simulink model "dynsim_edo"  (R2020a)
settings: Solver=ode3  StartTime=0.0  StopTime=10.0  FixedStep=0.001  RelTol=1e-3
model workspace (MAT data in the model file):
  SL_ROS_VariableLengthArrays_MaxSizes.CommonInfo.ArrayTruncateAction = 'EmitWarning'
  SL_ROS_VariableLengthArrays_MaxSizes.MsgTypeMap = containers.Map
  SL_ROS_VariableLengthArrays_MaxSizes.MsgTypeMap.serialization.keys = {}
  SL_ROS_VariableLengthArrays_MaxSizes.MsgTypeMap.serialization.values = {}
  SL_ROS_VariableLengthArrays_MaxSizes.MsgTypeMap.serialization.uniformity = 0
  SL_ROS_VariableLengthArrays_MaxSizes.MsgTypeMap.serialization.keyType = 'char'
  SL_ROS_VariableLengthArrays_MaxSizes.MsgTypeMap.serialization.valueType = 'any'
values from neighbouring files (symbols this model uses):
  L1 = 1    [init_edo.m]
  L2 = 1    [init_edo.m]
  L3 = 1    [init_edo.m]
  L4 = 1    [init_edo.m]
  L5 = 1    [init_edo.m]
  L6 = 1    [init_edo.m]
libraries: robotlib x18, robotmaniplib x1
settings Model: Creator=bascetta  LastModifiedBy=davide
settings OptimizationCC: EnhancedBackFolding=on  PassReuseOutputArgsAs=Individual arguments  ZeroExternalMemoryAtStartup=off  ZeroInternalMemoryAtStartup=off  MaxStackSize=64  OptimizeBlockOrder=speed  DifferentSizesBufferReuse=on  OptimizationCustomize=off  EfficientTunableParamExpr=on
settings DebuggingCC: ParameterTunabilityLossMsg=error
settings HardwareCC: ProdBitPerPointer=32  ProdBitPerSizeT=32  ProdBitPerPtrDiffT=32  ProdLargestAtomicFloat=None  ProdIntDivRoundTo=Undefined  ProdEndianess=Unspecified  ProdWordSize=32  ProdHWDeviceType=Generic->Unspecified (assume 32-bit Generic)
settings RTWCC: SystemTargetFile=ert.tlc  HardwareBoard=Robot Operating System (ROS)  TemplateMakefile=ert_default_tmf  GenerateReport=on  Toolchain=Catkin  IncludeHyperlinkInReport=on  LaunchReport=on  TargetLang=C++  GenerateTraceInfo=on  GenerateTraceReport=on  GenerateTraceReportSl=on  GenerateTraceReportSf=on  GenerateTraceReportEml=on
settings CodeAppCC: ForceParamTrailComments=on  IgnoreCustomStorageClasses=off  OperatorAnnotations=on  SimulinkDataObjDesc=on  SFDataObjDesc=on  InsertBlockDesc=on
settings ERTTargetCC: SupportContinuousTime=on  SupportVariableSizeSignals=on

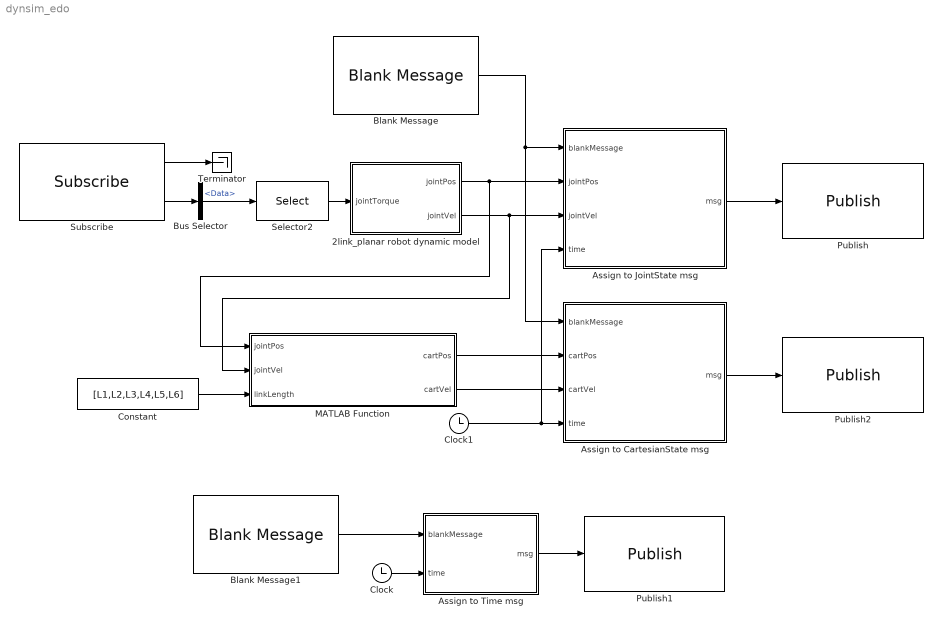
== system dynsim_edo ==
  2link_planar robot dynamic model : Subsystem
  Assign to CartesianState msg : MATLAB Function  TreatAsAtomicUnit=on
  Assign to JointState msg : MATLAB Function  TreatAsAtomicUnit=on
  Assign to Time msg : MATLAB Function  TreatAsAtomicUnit=on
  Blank Message : robotlib/Blank Message  messageClass=Message  entityType=sensor_msgs/JointState  messageType=sensor_msgs/JointState  SampleTime=inf
  Blank Message1 : robotlib/Blank Message  messageClass=Message  entityType=rosgraph_msgs/Clock  messageType=rosgraph_msgs/Clock  SampleTime=inf
  Bus Selector : BusSelector  OutputSignals=Data
  Clock : Clock
  Clock1 : Clock
  Constant : Constant  Value=[L1,L2,L3,L4,L5,L6]
  MATLAB Function : MATLAB Function  TreatAsAtomicUnit=on
  Publish : robotlib/Publish  topicSource=Specify your own  topic=/joint_states  messageType=sensor_msgs/JointState  messageQueueLength=1
  Publish1 : robotlib/Publish  topicSource=Specify your own  topic=/clock  messageType=rosgraph_msgs/Clock  messageQueueLength=1
  Publish2 : robotlib/Publish  topicSource=Specify your own  topic=/cartesian_states  messageType=sensor_msgs/JointState  messageQueueLength=1
  Selector2 : Selector  IndexOptions=Starting index (dialog)  Indices=[2]  OutputSizes=6
  Subscribe : robotlib/Subscribe  topicSource=Specify your own  topic=/joint_torque  messageType=std_msgs/Float64MultiArray  sampleTime=-1  messageQueueLength=1
  Terminator : Terminator
  wires:
  Blank Message1/1 -> Assign to Time msg/1(blankMessage)
  Assign to Time msg/1(msg) -> Publish1/1
  Subscribe/2 -> Bus Selector/1
  Subscribe/1 -> Terminator/1
  Selector2/1 -> 2link_planar robot dynamic model/1(jointTorque)
  Assign to JointState msg/1(msg) -> Publish/1
  2link_planar robot dynamic model/2(jointVel) -> MATLAB Function/2(jointVel), Assign to JointState msg/3(jointVel)
  Bus Selector/1 -> Selector2/1  "<Data>"
  2link_planar robot dynamic model/1(jointPos) -> MATLAB Function/1(jointPos), Assign to JointState msg/2(jointPos)
  Clock/1 -> Assign to Time msg/2(time)
  Clock1/1 -> Assign to CartesianState msg/4(time), Assign to JointState msg/4(time)
  MATLAB Function/2(cartVel) -> Assign to CartesianState msg/3(cartVel)
  Assign to CartesianState msg/1(msg) -> Publish2/1
  Constant/1 -> MATLAB Function/3(linkLength)
  MATLAB Function/1(cartPos) -> Assign to CartesianState msg/2(cartPos)
  Blank Message/1 -> Assign to CartesianState msg/1(blankMessage), Assign to JointState msg/1(blankMessage)

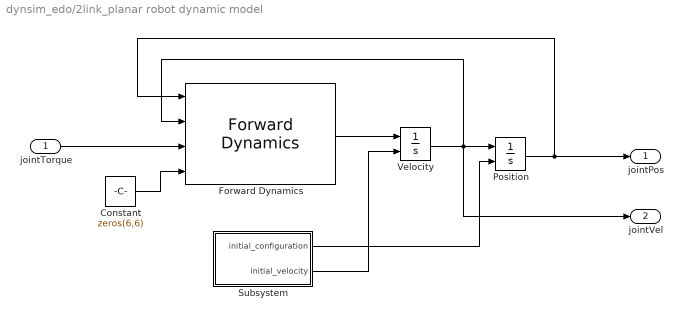
== system dynsim_edo/2link_planar robot dynamic model ==
  jointTorque : Inport
  Constant : Constant  Value=zeros(6,6)
  Forward Dynamics : robotmaniplib/Forward Dynamics  RigidBodyTree=robot_edo  SimulateUsing=Interpreted execution
  Position : Integrator  InitialConditionSource=external
  Subsystem : Subsystem
  Velocity : Integrator  InitialConditionSource=external
  jointPos : Outport
  jointVel : Outport  Port=2
  wires:
  Forward Dynamics/1 -> Velocity/1
  Position/1 -> Forward Dynamics/1, jointPos/1
  jointTorque/1 -> Forward Dynamics/3
  Constant/1 -> Forward Dynamics/4
  Velocity/1 -> Forward Dynamics/2, Position/1, jointVel/1
  Subsystem/2(initial_velocity) -> Velocity/2
  Subsystem/1(initial_configuration) -> Position/2

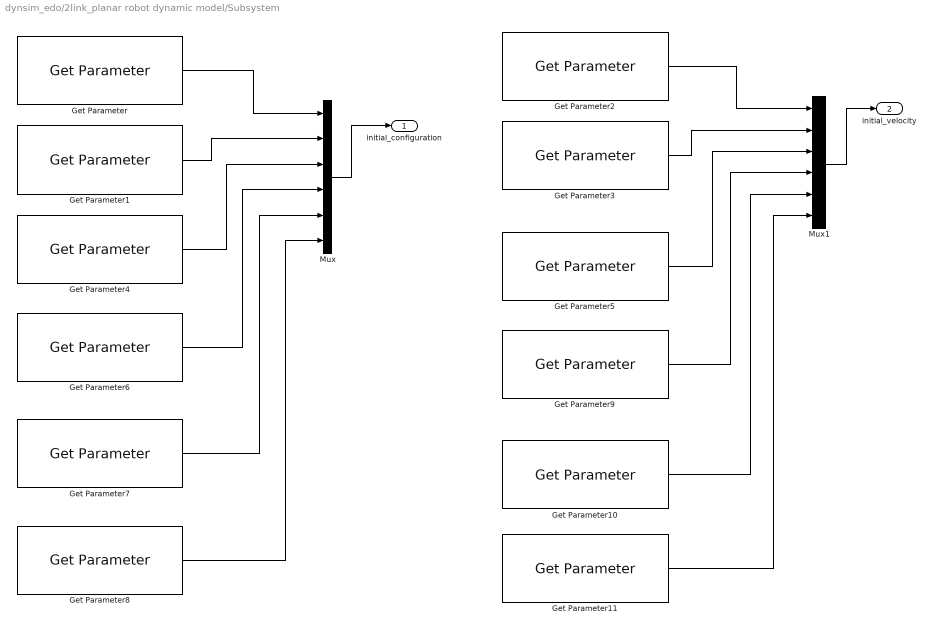
== system dynsim_edo/2link_planar robot dynamic model/Subsystem ==
  Get Parameter : robotlib/Get Parameter  ParameterSource=Specify your own  ParameterName=/dynsim_2link_planar/q1_initial  ParameterType=double  ParameterMaxArrayLength=16  ParameterInitialValue=pi/4  SampleTime=-1  ShowErrorCodeOutput=off  ModelName=dynsim_edo  BlockId=ParamGet_dynsim_edo_112
      settings: SourceProductBaseCode=RR
  Get Parameter1 : robotlib/Get Parameter  ParameterSource=Specify your own  ParameterName=/dynsim_2link_planar/q2_initial  ParameterType=double  ParameterMaxArrayLength=16  ParameterInitialValue=-pi/2  SampleTime=-1  ShowErrorCodeOutput=off  ModelName=dynsim_edo  BlockId=ParamGet_dynsim_edo_113
      settings: SourceProductBaseCode=RR
  Get Parameter10 : robotlib/Get Parameter  ParameterSource=Specify your own  ParameterName=/dynnsim_2link_planar/qv5_initial  ParameterType=double  ParameterMaxArrayLength=16  ParameterInitialValue=0  SampleTime=-1  ShowErrorCodeOutput=off  ModelName=dynsim_edo  BlockId=ParamGet_dynsim_edo_131
      settings: SourceProductBaseCode=RR
  Get Parameter11 : robotlib/Get Parameter  ParameterSource=Specify your own  ParameterName=/dynnsim_2link_planar/qv6_initial  ParameterType=double  ParameterMaxArrayLength=16  ParameterInitialValue=0  SampleTime=-1  ShowErrorCodeOutput=off  ModelName=dynsim_edo  BlockId=ParamGet_dynsim_edo_132
      settings: SourceProductBaseCode=RR
  Get Parameter2 : robotlib/Get Parameter  ParameterSource=Specify your own  ParameterName=/dynsim_2link_planar/qv1_initial  ParameterType=double  ParameterMaxArrayLength=16  ParameterInitialValue=0  SampleTime=-1  ShowErrorCodeOutput=off  ModelName=dynsim_edo  BlockId=ParamGet_dynsim_edo_117
      settings: SourceProductBaseCode=RR
  Get Parameter3 : robotlib/Get Parameter  ParameterSource=Specify your own  ParameterName=/dynnsim_2link_planar/qv2_initial  ParameterType=double  ParameterMaxArrayLength=16  ParameterInitialValue=0  SampleTime=-1  ShowErrorCodeOutput=off  ModelName=dynsim_edo  BlockId=ParamGet_dynsim_edo_118
      settings: SourceProductBaseCode=RR
  Get Parameter4 : robotlib/Get Parameter  ParameterSource=Specify your own  ParameterName=/dynsim_2link_planar/q3_initial  ParameterType=double  ParameterMaxArrayLength=16  ParameterInitialValue=-pi/2  SampleTime=-1  ShowErrorCodeOutput=off  ModelName=dynsim_edo  BlockId=ParamGet_dynsim_edo_125
      settings: SourceProductBaseCode=RR
  Get Parameter5 : robotlib/Get Parameter  ParameterSource=Specify your own  ParameterName=/dynnsim_2link_planar/qv3_initial  ParameterType=double  ParameterMaxArrayLength=16  ParameterInitialValue=0  SampleTime=-1  ShowErrorCodeOutput=off  ModelName=dynsim_edo  BlockId=ParamGet_dynsim_edo_126
      settings: SourceProductBaseCode=RR
  Get Parameter6 : robotlib/Get Parameter  ParameterSource=Specify your own  ParameterName=/dynsim_2link_planar/q4_initial  ParameterType=double  ParameterMaxArrayLength=16  ParameterInitialValue=-pi/2  SampleTime=-1  ShowErrorCodeOutput=off  ModelName=dynsim_edo  BlockId=ParamGet_dynsim_edo_127
      settings: SourceProductBaseCode=RR
  Get Parameter7 : robotlib/Get Parameter  ParameterSource=Specify your own  ParameterName=/dynsim_2link_planar/q5_initial  ParameterType=double  ParameterMaxArrayLength=16  ParameterInitialValue=-pi/2  SampleTime=-1  ShowErrorCodeOutput=off  ModelName=dynsim_edo  BlockId=ParamGet_dynsim_edo_128
      settings: SourceProductBaseCode=RR
  Get Parameter8 : robotlib/Get Parameter  ParameterSource=Specify your own  ParameterName=/dynsim_2link_planar/q6_initial  ParameterType=double  ParameterMaxArrayLength=16  ParameterInitialValue=-pi/2  SampleTime=-1  ShowErrorCodeOutput=off  ModelName=dynsim_edo  BlockId=ParamGet_dynsim_edo_129
      settings: SourceProductBaseCode=RR
  Get Parameter9 : robotlib/Get Parameter  ParameterSource=Specify your own  ParameterName=/dynnsim_2link_planar/qv4_initial  ParameterType=double  ParameterMaxArrayLength=16  ParameterInitialValue=0  SampleTime=-1  ShowErrorCodeOutput=off  ModelName=dynsim_edo  BlockId=ParamGet_dynsim_edo_130
      settings: SourceProductBaseCode=RR
  Mux : Mux  Inputs=6
  Mux1 : Mux  Inputs=6
  initial_configuration : Outport
  initial_velocity : Outport  Port=2
  wires:
  Mux/1 -> initial_configuration/1
  Get Parameter/1 -> Mux/1
  Get Parameter1/1 -> Mux/2
  Get Parameter3/1 -> Mux1/2
  Get Parameter2/1 -> Mux1/1
  Mux1/1 -> initial_velocity/1
  Get Parameter4/1 -> Mux/3
  Get Parameter5/1 -> Mux1/3
  Get Parameter6/1 -> Mux/4
  Get Parameter7/1 -> Mux/5
  Get Parameter8/1 -> Mux/6
  Get Parameter9/1 -> Mux1/4
  Get Parameter10/1 -> Mux1/5
  Get Parameter11/1 -> Mux1/6

== matlab function dynsim_edo/Assign to Time msg ==
  data: blankMessage input; msg output Bus: SL_Bus_dynsim_edo_rosgraph_msgs_Clock; time input
function msg = assign_Time(blankMessage,time)
%#codegen

% Assign the output message to be the same with input blank message
msg = blankMessage;

% Convert and set time
msg.Clock_.Sec  = fix(time);
msg.Clock_.Nsec = fix((time-fix(time))*1e9);

== matlab function dynsim_edo/Assign to JointState msg ==
  data: blankMessage input; msg output Bus: SL_Bus_dynsim_edo_sensor_msgs_JointState; jointPos input; jointVel input; time input
function msg = assign_JointState(blankMessage,jointPos,jointVel,time)
%#codegen

% Assign the output message to be the same with input blank message
msg = blankMessage;

% Initialize time stamp
msg.Header.Stamp.Sec  = fix(time);
msg.Header.Stamp.Nsec = fix((time-fix(time))*1e9);

% Set the number of strings in the string array, and joint positions/velocities in the position/velocity array
numJoints = length(jointPos);
msg.Name_SL_Info.CurrentLength = uint32(numJoints);
msg.Position_SL_Info.CurrentLength = uint32(numJoints);
msg.Velocity_SL_Info.CurrentLength = uint32(numJoints);

% Set the individual components in the message arrays
strArrayToAssign = {'joint_1', 'joint_2','joint_3','joint_4','joint_5','joint_6'};

for idx=1:numJoints
    str = strArrayToAssign{idx};
    strLength = length(str);
    msg.Name(idx).Data(1:strLength) = uint8(str);
    msg.Name(idx).Data_SL_Info.CurrentLength = uint32(strLength);

    msg.Position(idx) = jointPos(idx);
    msg.Velocity(idx) = jointVel(idx);
end

== matlab function dynsim_edo/MATLAB Function ==
  data: jointPos input; cartPos output; jointVel input; cartVel output; linkLength input
function [cartPos, cartVel] = forward_kinematics_2link(jointPos,jointVel,linkLength)

cartPos = zeros(1,2);
cartVel = zeros(1,2);

L1 = linkLength(1);
L2 = linkLength(2);
L3 = linkLength(3);
L4 = linkLength(4);
L5 = linkLength(5);
L6 = linkLength(6);
q1 = jointPos(1);
q2 = jointPos(2);
q3 = jointPos(3);
q4 = jointPos(4);
q5 = jointPos(5);
q6 = jointPos(6);
qv1 = jointVel(1);
qv2 = jointVel(2);
qv3 = jointVel(3);
qv4 = jointVel(4);
qv5 = jointVel(5);
qv6 = jointVel(6);

cartPos(1) = L1*cos(q1)+L2*cos(q1+q2)+L3*cos(q1+q2+q3)+L4*cos(q1+q2+q3+q4)+L5*cos(q1+q2+q3+q4+q5)+L6*cos(q1+q2+q3+q4+q5+q6);
cartPos(2) = L1*sin(q1)+L2*sin(q1+q2)+L3*sin(q1+q2+q3)+L4*sin(q1+q2+q3+q4)+L5*sin(q1+q2+q3+q4+q5)+L6*sin(q1+q2+q3+q4+q5+q6);
cartVel(1) = -L1*qv1*sin(q1)-L2*(qv1+qv2)*sin(q1+q2)-L3*(qv1+qv2+qv3)*sin(q1+q2+q3)-L4*(qv1+qv2+qv3+qv4)*sin(q1+q2+q3+q4)-L5*(qv1+qv2+qv3+qv4+qv5)*sin(q1+q2+q3+q4+q5)-L6*(qv1+qv2+qv3+qv4+qv5+qv6)*sin(q1+q2+q3+q4+q5+q6);
cartVel(2) = L1*qv1*cos(q1)+L2*(qv1+qv2)*cos(q1+q2)+L3*(qv1+qv2+qv3)*cos(q1+q2+q3)+L4*(qv1+qv2+qv3+qv4)*cos(q1+q2+q3+q4)+L5*(qv1+qv2+qv3+qv4+qv5)*cos(q1+q2+q3+q4+q5)+L6*(qv1+qv2+qv3+qv4+qv5+qv6)*cos(q1+q2+q3+q4+q5+q6);

== matlab function dynsim_edo/Assign to CartesianState msg ==
  data: blankMessage input; msg output Bus: SL_Bus_dynsim_edo_sensor_msgs_JointState; cartPos input; cartVel input; time input
function msg = assign_CartesianState(blankMessage,cartPos,cartVel,time)
%#codegen

% Assign the output message to be the same with input blank message
msg = blankMessage;

% Initialize time stamp
msg.Header.Stamp.Sec  = fix(time);
msg.Header.Stamp.Nsec = fix((time-fix(time))*1e9);

% Set the number of strings in the string array, and Cartesian positions/velocities
% in the position/velocity array
numCoordinates = length(cartPos);
msg.Name_SL_Info.CurrentLength = uint32(numCoordinates);
msg.Position_SL_Info.CurrentLength = uint32(numCoordinates);
msg.Velocity_SL_Info.CurrentLength = uint32(numCoordinates);

% Set the individual components in the message arrays
strArrayToAssign = {'joint_1', 'joint_2','joint_3','joint_4','joint_5','joint_6'};

for idx=1:numCoordinates
    str = strArrayToAssign{idx};
    strLength = length(str);
    msg.Name(idx).Data(1:strLength) = uint8(str);
    msg.Name(idx).Data_SL_Info.CurrentLength = uint32(strLength);

    msg.Position(idx) = cartPos(idx);
    msg.Velocity(idx) = cartVel(idx);
end
